simulink model "Pacemaker_model_2018b"  (R2018b)
settings: Solver=FixedStepAuto  StartTime=0.0  StopTime=inf  FixedStep=1e-3  RelTol=1e-3  EnableMultiTasking=on
undefined symbols (not defined in the file): D0, D1, D10, D11, D12, D13, D2, D3, D4, D5, D6, D7, D8, D9, PTA0, PTA1, PTA2, PTB23, PTB9, PTC16, PTC17, PTC2, PTC3, PTC4, PTD0, PTD1, PTD2, PTD3
libraries: frdmk64flib x18
settings Model: ExtModeTrigDuration=5  Creator=dr_pa  LastModifiedBy=dr_pa
settings DataIOCC: ReturnWorkspaceOutputs=on
settings OptimizationCC: EnhancedBackFolding=on  PassReuseOutputArgsAs=Individual arguments  MaxStackSize=64  OptimizeBlockOrder=speed  DifferentSizesBufferReuse=on  OptimizationCustomize=off
settings DebuggingCC: ParameterTunabilityLossMsg=error
settings HardwareCC: ProdBitPerPointer=32  ProdBitPerSizeT=32  ProdBitPerPtrDiffT=32  ProdLargestAtomicInteger=Long  ProdLargestAtomicFloat=Double  ProdWordSize=32  ProdHWDeviceType=ARM Compatible->ARM Cortex
settings SFSimCC: MATLABDynamicMemAlloc=off
settings RTWCC: SystemTargetFile=ert.tlc  HardwareBoard=NXP FRDM-K64F  TLCOptions="-aInlineSetEventsForThisBaseRateFcn=TLC_FALSE -aSuppressMultiTaskScheduler=TLC_FALSE  -aRateBasedStepFcn=0"  TemplateMakefile=ert_default_tmf  GenerateReport=on  Toolchain=GNU Tools for ARM Embedded Processors  IncludeHyperlinkInReport=on  LaunchReport=on  GenerateTraceInfo=on  GenerateTraceReport=on  GenerateTraceReportSl=on  GenerateTraceReportSf=on  GenerateTraceReportEml=on
settings CodeAppCC: ForceParamTrailComments=on  IgnoreCustomStorageClasses=off  OperatorAnnotations=on  SimulinkDataObjDesc=on  SFDataObjDesc=on  InsertBlockDesc=on

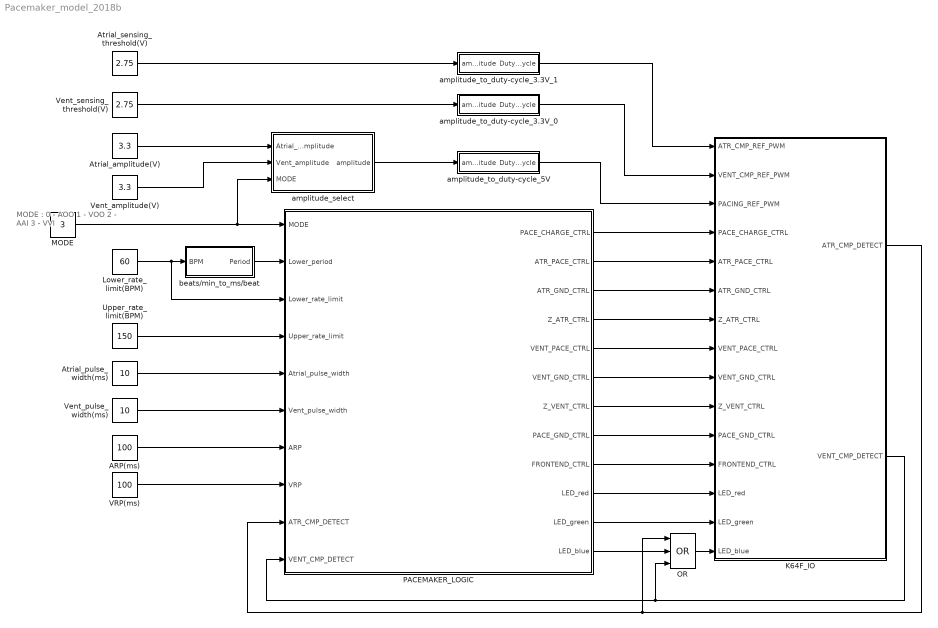
== system Pacemaker_model_2018b ==
  note: MODE :
      | 0 - AOO
      | 1 - VOO
      | 2 - AAI
      | 3 - VVI
  ARP(ms) : Constant  Value=100  OutDataTypeStr=uint16
  Atrial_amplitude(V) : Constant  Value=3.3  OutDataTypeStr=double
  Atrial_pulse_width(ms) : Constant  Value=10  OutDataTypeStr=uint16
  Atrial_sensing_threshold(V) : Constant  Value=2.75  OutDataTypeStr=double
  K64F_IO : Subsystem
  Lower_rate_limit(BPM) : Constant  Value=60  OutDataTypeStr=uint16
  MODE : Constant  Value=3  OutDataTypeStr=uint8
  OR : Logic  Operator=OR  Inputs=3  IconShape=distinctive  AllPortsSameDT=off  OutDataTypeStr=boolean
  PACEMAKER_LOGIC : Stateflow chart  TreatAsAtomicUnit=on
  Upper_rate_limit(BPM) : Constant  Value=150  OutDataTypeStr=uint16
  VRP(ms) : Constant  Value=100  OutDataTypeStr=uint16
  Vent_amplitude(V) : Constant  Value=3.3  OutDataTypeStr=double
  Vent_pulse_width(ms) : Constant  Value=10  OutDataTypeStr=uint16
  Vent_sensing_threshold(V) : Constant  Value=2.75  OutDataTypeStr=double
  amplitude_select : Subsystem
  amplitude_to_duty-cycle_3.3V_0 : Subsystem
  amplitude_to_duty-cycle_3.3V_1 : Subsystem
  amplitude_to_duty-cycle_5V : Subsystem
  beats/min_to_ms/beat : Subsystem
  wires:
  Atrial_pulse_width(ms)/1 -> PACEMAKER_LOGIC/5(Atrial_pulse_width)
  MODE/1 -> amplitude_select/3(MODE), PACEMAKER_LOGIC/1(MODE)
  PACEMAKER_LOGIC/8(PACE_GND_CTRL) -> K64F_IO/11(PACE_GND_CTRL)
  PACEMAKER_LOGIC/7(Z_VENT_CTRL) -> K64F_IO/10(Z_VENT_CTRL)
  PACEMAKER_LOGIC/6(VENT_GND_CTRL) -> K64F_IO/9(VENT_GND_CTRL)
  PACEMAKER_LOGIC/5(VENT_PACE_CTRL) -> K64F_IO/8(VENT_PACE_CTRL)
  PACEMAKER_LOGIC/4(Z_ATR_CTRL) -> K64F_IO/7(Z_ATR_CTRL)
  PACEMAKER_LOGIC/3(ATR_GND_CTRL) -> K64F_IO/6(ATR_GND_CTRL)
  PACEMAKER_LOGIC/2(ATR_PACE_CTRL) -> K64F_IO/5(ATR_PACE_CTRL)
  PACEMAKER_LOGIC/1(PACE_CHARGE_CTRL) -> K64F_IO/4(PACE_CHARGE_CTRL)
  amplitude_to_duty-cycle_5V/1(Duty Cycle) -> K64F_IO/3(PACING_REF_PWM)
  Vent_pulse_width(ms)/1 -> PACEMAKER_LOGIC/6(Vent_pulse_width)
  Lower_rate_limit(BPM)/1 -> PACEMAKER_LOGIC/3(Lower_rate_limit), beats/min_to_ms/beat/1(BPM)
  beats/min_to_ms/beat/1(Period) -> PACEMAKER_LOGIC/2(Lower_period)
  Upper_rate_limit(BPM)/1 -> PACEMAKER_LOGIC/4(Upper_rate_limit)
  amplitude_select/1(amplitude) -> amplitude_to_duty-cycle_5V/1(amplitude)
  Vent_amplitude(V)/1 -> amplitude_select/2(Vent_amplitude)
  Atrial_amplitude(V)/1 -> amplitude_select/1(Atrial_amplitude)
  amplitude_to_duty-cycle_3.3V_0/1(Duty Cycle) -> K64F_IO/2(VENT_CMP_REF_PWM)
  Vent_sensing_threshold(V)/1 -> amplitude_to_duty-cycle_3.3V_0/1(amplitude)
  Atrial_sensing_threshold(V)/1 -> amplitude_to_duty-cycle_3.3V_1/1(amplitude)
  amplitude_to_duty-cycle_3.3V_1/1(Duty Cycle) -> K64F_IO/1(ATR_CMP_REF_PWM)
  PACEMAKER_LOGIC/9(FRONTEND_CTRL) -> K64F_IO/12(FRONTEND_CTRL)
  ARP(ms)/1 -> PACEMAKER_LOGIC/7(ARP)
  VRP(ms)/1 -> PACEMAKER_LOGIC/8(VRP)
  PACEMAKER_LOGIC/11(LED_green) -> K64F_IO/14(LED_green)
  K64F_IO/1(ATR_CMP_DETECT) -> PACEMAKER_LOGIC/9(ATR_CMP_DETECT), OR/1
  K64F_IO/2(VENT_CMP_DETECT) -> OR/3, PACEMAKER_LOGIC/10(VENT_CMP_DETECT)
  PACEMAKER_LOGIC/10(LED_red) -> K64F_IO/13(LED_red)
  OR/1 -> K64F_IO/15(LED_blue)
  PACEMAKER_LOGIC/12(LED_blue) -> OR/2

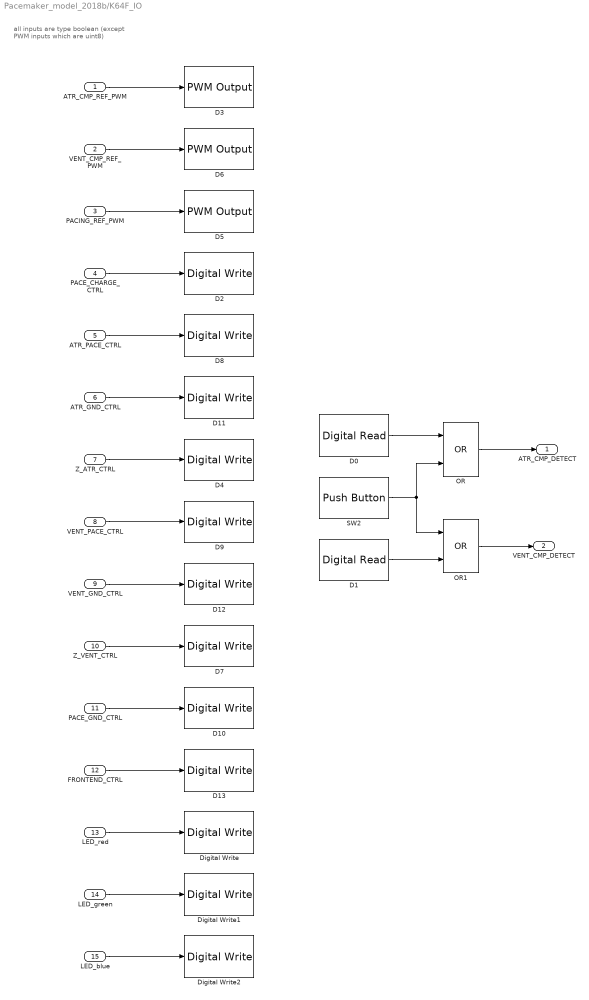
== system Pacemaker_model_2018b/K64F_IO ==
  note: all inputs are type boolean
      | (except PWM inputs which are uint8)
  ATR_CMP_REF_PWM : Inport  OutDataTypeStr=uint8
  VENT_CMP_REF_PWM : Inport  Port=2  OutDataTypeStr=uint8
  PACING_REF_PWM : Inport  Port=3  OutDataTypeStr=uint8
  PACE_CHARGE_CTRL : Inport  Port=4  OutDataTypeStr=boolean
  ATR_PACE_CTRL : Inport  Port=5  OutDataTypeStr=boolean
  ATR_GND_CTRL : Inport  Port=6  OutDataTypeStr=boolean
  Z_ATR_CTRL : Inport  Port=7  OutDataTypeStr=boolean
  VENT_PACE_CTRL : Inport  Port=8  OutDataTypeStr=boolean
  VENT_GND_CTRL : Inport  Port=9  OutDataTypeStr=boolean
  Z_VENT_CTRL : Inport  Port=10  OutDataTypeStr=boolean
  PACE_GND_CTRL : Inport  Port=11  OutDataTypeStr=boolean
  FRONTEND_CTRL : Inport  Port=12  OutDataTypeStr=boolean
  LED_red : Inport  Port=13  OutDataTypeStr=boolean
  LED_green : Inport  Port=14  OutDataTypeStr=boolean
  LED_blue : Inport  Port=15  OutDataTypeStr=boolean
  D0 : frdmk64flib/Digital Read  Whichpin=PTC16 (D0)  SampleTime=-1
      settings: SourceProductName=Simulink Coder Support Package for NXP FRDM-K64F Board
  D1 : frdmk64flib/Digital Read  Whichpin=PTC17 (D1)  SampleTime=-1
      settings: SourceProductName=Simulink Coder Support Package for NXP FRDM-K64F Board
  D10 : frdmk64flib/Digital Write  Whichpin=PTD0 (D10)
      settings: SourceProductName=Simulink Coder Support Package for NXP FRDM-K64F Board
  D11 : frdmk64flib/Digital Write  Whichpin=PTD2 (D11)
      settings: SourceProductName=Simulink Coder Support Package for NXP FRDM-K64F Board
  D12 : frdmk64flib/Digital Write  Whichpin=PTD3 (D12)
      settings: SourceProductName=Simulink Coder Support Package for NXP FRDM-K64F Board
  D13 : frdmk64flib/Digital Write  Whichpin=PTD1 (D13)
      settings: SourceProductName=Simulink Coder Support Package for NXP FRDM-K64F Board
  D2 : frdmk64flib/Digital Write  Whichpin=PTB9 (D2)
      settings: SourceProductName=Simulink Coder Support Package for NXP FRDM-K64F Board
  D3 : frdmk64flib/PWM Output  Whichpin=PTA1 (D3)  InitialFrequency=2000  InitialDutyCycle=0
      settings: SourceProductName=Simulink Coder Support Package for NXP FRDM-K64F Board
  D4 : frdmk64flib/Digital Write  Whichpin=PTB23 (D4)
      settings: SourceProductName=Simulink Coder Support Package for NXP FRDM-K64F Board
  D5 : frdmk64flib/PWM Output  Whichpin=PTA2 (D5)  InitialFrequency=2000  InitialDutyCycle=0
      settings: SourceProductName=Simulink Coder Support Package for NXP FRDM-K64F Board
  D6 : frdmk64flib/PWM Output  Whichpin=PTC2 (D6)  InitialFrequency=2000  InitialDutyCycle=0
      settings: SourceProductName=Simulink Coder Support Package for NXP FRDM-K64F Board
  D7 : frdmk64flib/Digital Write  Whichpin=PTC3 (D7)
      settings: SourceProductName=Simulink Coder Support Package for NXP FRDM-K64F Board
  D8 : frdmk64flib/Digital Write  Whichpin=PTA0 (D8)
      settings: SourceProductName=Simulink Coder Support Package for NXP FRDM-K64F Board
  D9 : frdmk64flib/Digital Write  Whichpin=PTC4 (D9)
      settings: SourceProductName=Simulink Coder Support Package for NXP FRDM-K64F Board
  Digital Write : frdmk64flib/Digital Write  Whichpin=RED_LED
      settings: SourceProductName=Simulink Coder Support Package for NXP FRDM-K64F Board
  Digital Write1 : frdmk64flib/Digital Write  Whichpin=GREEN_LED
      settings: SourceProductName=Simulink Coder Support Package for NXP FRDM-K64F Board
  Digital Write2 : frdmk64flib/Digital Write  Whichpin=BLUE_LED
      settings: SourceProductName=Simulink Coder Support Package for NXP FRDM-K64F Board
  OR : Logic  Operator=OR  IconShape=distinctive  AllPortsSameDT=off  OutDataTypeStr=boolean
  OR1 : Logic  Operator=OR  IconShape=distinctive  AllPortsSameDT=off  OutDataTypeStr=boolean
  SW2 : frdmk64flib/Push Button  Whichswitch=SW2  SampleTime1=-1
      settings: SourceProductName=Simulink Coder Support Package for NXP FRDM-K64F Board
  ATR_CMP_DETECT : Outport  OutDataTypeStr=boolean
  VENT_CMP_DETECT : Outport  Port=2  OutDataTypeStr=boolean
  wires:
  PACING_REF_PWM/1 -> D5/1
  PACE_CHARGE_CTRL/1 -> D2/1
  VENT_PACE_CTRL/1 -> D9/1
  VENT_GND_CTRL/1 -> D12/1
  ATR_PACE_CTRL/1 -> D8/1
  ATR_GND_CTRL/1 -> D11/1
  PACE_GND_CTRL/1 -> D10/1
  Z_ATR_CTRL/1 -> D4/1
  Z_VENT_CTRL/1 -> D7/1
  FRONTEND_CTRL/1 -> D13/1
  ATR_CMP_REF_PWM/1 -> D3/1
  VENT_CMP_REF_PWM/1 -> D6/1
  LED_red/1 -> Digital Write/1
  LED_green/1 -> Digital Write1/1
  D0/1 -> OR/1
  D1/1 -> OR1/2
  SW2/1 -> OR/2, OR1/1
  OR/1 -> ATR_CMP_DETECT/1
  OR1/1 -> VENT_CMP_DETECT/1
  LED_blue/1 -> Digital Write2/1

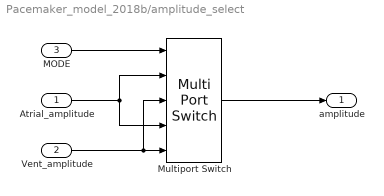
== system Pacemaker_model_2018b/amplitude_select ==
  Atrial_amplitude : Inport  OutDataTypeStr=double
  Vent_amplitude : Inport  Port=2  OutDataTypeStr=double
  MODE : Inport  Port=3  OutDataTypeStr=uint8
  Multiport Switch : MultiPortSwitch  DataPortOrder=Zero-based contiguous  Inputs=4  zeroidx=on
  amplitude : Outport  OutDataTypeStr=double
  wires:
  Multiport Switch/1 -> amplitude/1
  MODE/1 -> Multiport Switch/1
  Atrial_amplitude/1 -> Multiport Switch/4, Multiport Switch/2
  Vent_amplitude/1 -> Multiport Switch/5, Multiport Switch/3

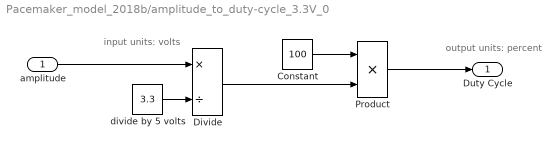
== system Pacemaker_model_2018b/amplitude_to_duty-cycle_3.3V_0 ==
  note: input units: volts
  note: output units: percent
  amplitude : Inport  OutDataTypeStr=double
  Constant : Constant  Value=100  OutDataTypeStr=double
  Divide : Product  Inputs=*/  OutDataTypeStr=double
  Product : Product  OutDataTypeStr=uint8  RndMeth=Round
  divide by 5 volts : Constant  Value=3.3  OutDataTypeStr=double
  Duty Cycle : Outport  OutDataTypeStr=uint8
  wires:
  amplitude/1 -> Divide/1
  Product/1 -> Duty Cycle/1
  Constant/1 -> Product/1
  Divide/1 -> Product/2
  divide by 5 volts/1 -> Divide/2

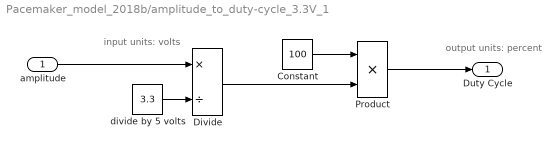
== system Pacemaker_model_2018b/amplitude_to_duty-cycle_3.3V_1 ==
  note: output units: percent
  note: input units: volts
  amplitude : Inport  OutDataTypeStr=double
  Constant : Constant  Value=100  OutDataTypeStr=double
  Divide : Product  Inputs=*/  OutDataTypeStr=double
  Product : Product  OutDataTypeStr=uint8  RndMeth=Round
  divide by 5 volts : Constant  Value=3.3  OutDataTypeStr=double
  Duty Cycle : Outport  OutDataTypeStr=uint8
  wires:
  divide by 5 volts/1 -> Divide/2
  Divide/1 -> Product/2
  Constant/1 -> Product/1
  Product/1 -> Duty Cycle/1
  amplitude/1 -> Divide/1

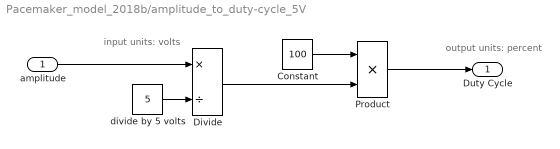
== system Pacemaker_model_2018b/amplitude_to_duty-cycle_5V ==
  note: output units: percent
  note: input units: volts
  amplitude : Inport  OutDataTypeStr=double
  Constant : Constant  Value=100  OutDataTypeStr=double
  Divide : Product  Inputs=*/  OutDataTypeStr=double
  Product : Product  OutDataTypeStr=uint8  RndMeth=Round
  divide by 5 volts : Constant  Value=5  OutDataTypeStr=double
  Duty Cycle : Outport  OutDataTypeStr=uint8
  wires:
  divide by 5 volts/1 -> Divide/2
  Divide/1 -> Product/2
  Constant/1 -> Product/1
  Product/1 -> Duty Cycle/1
  amplitude/1 -> Divide/1

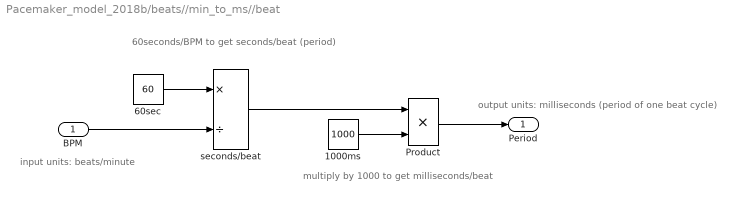
== system Pacemaker_model_2018b/beats//min_to_ms//beat ==
  note: input units: beats/minute
  note: output units: milliseconds (period of one beat cycle)
  note: 60seconds/BPM to get seconds/beat (period)
  note: multiply by 1000 to get milliseconds/beat
  BPM : Inport  OutDataTypeStr=uint16
  1000ms : Constant  Value=1000  OutDataTypeStr=double
  60sec : Constant  Value=60  OutDataTypeStr=double
  Product : Product  OutDataTypeStr=uint16  RndMeth=Round
  seconds/beat : Product  Inputs=*/  OutDataTypeStr=double
  Period : Outport  OutDataTypeStr=uint16
  wires:
  1000ms/1 -> Product/2
  Product/1 -> Period/1
  seconds/beat/1 -> Product/1
  60sec/1 -> seconds/beat/1
  BPM/1 -> seconds/beat/2

== stateflow chart Pacemaker_model_2018b/PACEMAKER_LOGIC ==
  state AOO [group]
    state AOO_PACE_ATRIUM
      entry:
      LED_green = true;
      PACE_CHARGE_CTRL = false;
      PACE_GND_CTRL = true;
      VENT_PACE_CTRL = false;
      VENT_GND_CTRL = false;
      Z_VENT_CTRL = false;
      Z_ATR_CTRL = false;
      ATR_GND_CTRL = false;
      ATR_PACE_CTRL = true;
    state AOO_DischargeC21_ChargeC22
      entry:
      LED_red = false;
      LED_green = false;
      PACE_GND_CTRL = true;
      ATR_PACE_CTRL = false;
      Z_ATR_CTRL = false;
      Z_VENT_CTRL = false;
      VENT_PACE_CTRL = false;
      VENT_GND_CTRL = false;
      ATR_GND_CTRL = true;
      PACE_CHARGE_CTRL = true;
    AOO_DischargeC21_ChargeC22 -> AOO_PACE_ATRIUM : after((Lower_period-Atrial_pulse_width), msec)
    AOO_PACE_ATRIUM -> AOO_DischargeC21_ChargeC22 : after(Atrial_pulse_width, msec)
  state VOO [group]
    state VOO_PACE_VENT
      entry:
      LED_green = true;
      PACE_CHARGE_CTRL = false;
      PACE_GND_CTRL = true;
      ATR_PACE_CTRL = false;
      ATR_GND_CTRL = false;
      Z_ATR_CTRL = false;
      Z_VENT_CTRL = false;
      VENT_GND_CTRL = false;
      VENT_PACE_CTRL = true;
    state VOO_DischargeC21_ChargeC22
      entry:
      LED_red = false;
      LED_green = false;
      PACE_GND_CTRL = true;
      VENT_PACE_CTRL = false;
      Z_VENT_CTRL = false;
      Z_ATR_CTRL = false;
      ATR_PACE_CTRL = false;
      ATR_GND_CTRL = false;
      VENT_GND_CTRL = true;
      PACE_CHARGE_CTRL = true;
    VOO_DischargeC21_ChargeC22 -> VOO_PACE_VENT : after((Lower_period-Vent_pulse_width), msec)
    VOO_PACE_VENT -> VOO_DischargeC21_ChargeC22 : after(Vent_pulse_width, msec)
  state HOLD
    entry:
    PACE_CHARGE_CTRL = false;
    PACE_GND_CTRL = false;
    ATR_GND_CTRL = false;
    VENT_GND_CTRL = false;
    ATR_PACE_CTRL = false;
    VENT_PACE_CTRL = false;
    FRONTEND_CTRL = true;
    LED_red = true;
    LED_green = false;
    LED_blue = false;
  state AAI [group]
    state ARP
      entry:
      LED_green = false;
      PACE_GND_CTRL = true;
      ATR_PACE_CTRL = false;
      Z_ATR_CTRL = false;
      Z_VENT_CTRL = false;
      VENT_PACE_CTRL = false;
      VENT_GND_CTRL = false;
      ATR_GND_CTRL = true;
      PACE_CHARGE_CTRL = true;
    state AAI_PACE_ATRIUM
      entry:
      FRONTEND_CTRL = false;
      LED_green = true;
      PACE_CHARGE_CTRL = false;
      PACE_GND_CTRL = true;
      VENT_PACE_CTRL = false;
      VENT_GND_CTRL = false;
      Z_VENT_CTRL = false;
      Z_ATR_CTRL = false;
      ATR_GND_CTRL = false;
      ATR_PACE_CTRL = true;
    state AAI_DischargeC21_ChargeC22
      entry:
      FRONTEND_CTRL = true;
      LED_blue = false;
      LED_red = false;
      LED_green = false;
      PACE_GND_CTRL = true;
      ATR_PACE_CTRL = false;
      Z_ATR_CTRL = false;
      Z_VENT_CTRL = false;
      VENT_PACE_CTRL = false;
      VENT_GND_CTRL = false;
      ATR_GND_CTRL = true;
      PACE_CHARGE_CTRL = true;
    AAI_PACE_ATRIUM -> ARP : after(Atrial_pulse_width, msec)
    AAI_DischargeC21_ChargeC22 -> ARP [order 1] : [ATR_CMP_DETECT==true]
    ARP -> AAI_DischargeC21_ChargeC22 : after(ARP, msec)
    AAI_DischargeC21_ChargeC22 -> AAI_PACE_ATRIUM [order 2] : after((Lower_period-Atrial_pulse_width-ARP), msec)
  state VVI [group]
    state VRP
      entry:
      LED_green = false;
      PACE_GND_CTRL = true;
      VENT_PACE_CTRL = false;
      Z_VENT_CTRL = false;
      Z_ATR_CTRL = false;
      ATR_PACE_CTRL = false;
      ATR_GND_CTRL = false;
      VENT_GND_CTRL = true;
      PACE_CHARGE_CTRL = true;
    state VVI_PACE_VENT
      entry:
      FRONTEND_CTRL = false;
      LED_green = true;
      PACE_CHARGE_CTRL = false;
      PACE_GND_CTRL = true;
      ATR_PACE_CTRL = false;
      ATR_GND_CTRL = false;
      Z_ATR_CTRL = false;
      Z_VENT_CTRL = false;
      VENT_GND_CTRL = false;
      VENT_PACE_CTRL = true;
    state VVI_DischargeC21_ChargeC22
      entry:
      FRONTEND_CTRL = true;
      LED_blue = false;
      LED_red = false;
      LED_green = false;
      PACE_GND_CTRL = true;
      VENT_PACE_CTRL = false;
      Z_VENT_CTRL = false;
      Z_ATR_CTRL = false;
      ATR_PACE_CTRL = false;
      ATR_GND_CTRL = false;
      VENT_GND_CTRL = true;
      PACE_CHARGE_CTRL = true;
    VVI_DischargeC21_ChargeC22 -> VRP [order 1] : [VENT_CMP_DETECT==true]
    VVI_PACE_VENT -> VRP : after(Vent_pulse_width, msec)
    VRP -> VVI_DischargeC21_ChargeC22 : after(VRP, msec)
    VVI_DischargeC21_ChargeC22 -> VVI_PACE_VENT [order 2] : after(Lower_period-Vent_pulse_width-ARP, msec)
  HOLD -> AAI_DischargeC21_ChargeC22 [order 3] : [MODE==2]
  HOLD -> VOO_DischargeC21_ChargeC22 [order 4] : [MODE==1]
  HOLD -> AOO_DischargeC21_ChargeC22 [order 2] : [MODE==0]
  (default) -> HOLD
  HOLD -> HOLD [order 1] : [Lower_rate_limit>Upper_rate_limit]
  HOLD -> VVI_DischargeC21_ChargeC22 [order 5] : [MODE==3]
  data: MODE input uint8; Lower_period input uint16; Lower_rate_limit input uint16; Upper_rate_limit input uint16; Atrial_pulse_width input uint16; PACE_CHARGE_CTRL output boolean; ATR_PACE_CTRL output boolean; ATR_GND_CTRL output boolean; Z_ATR_CTRL output boolean; VENT_PACE_CTRL output boolean; VENT_GND_CTRL output boolean; Z_VENT_CTRL output boolean; PACE_GND_CTRL output boolean; FRONTEND_CTRL output boolean; LED_red output boolean; LED_green output boolean; LED_blue output boolean; Vent_pulse_width input uint16; ARP input uint16; VRP input uint16; ATR_CMP_DETECT input boolean; VENT_CMP_DETECT input boolean
